simulink model "SignalRouting_Demo"  (R2017b)
settings: Solver=VariableStepAuto  StartTime=0.0  StopTime=10.0  RelTol=1e-3
settings Model: Creator=javed  LastModifiedBy=javed

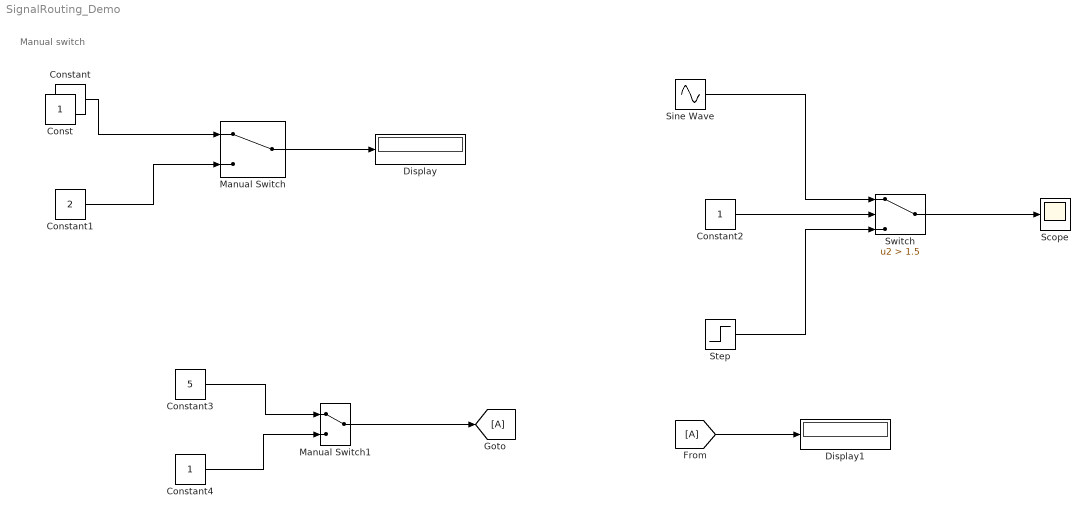
== system SignalRouting_Demo ==
  note: Manual switch
  Constant : Constant  Value=5
  Constant1 : Constant  Value=2
  Constant2 : Constant
  Constant3 : Constant  Value=5
  Constant4 : Constant
  Display : Display
  Display1 : Display
  Manual Switch : ManualSwitch
  Manual Switch1 : ManualSwitch
  Scope : Scope
  Sine Wave : Sin  SampleTime=0
  Step : Step  After=2  SampleTime=0
  Switch : Switch  Criteria=u2 > Threshold  Threshold=1.5
  Const : Constant  IOType=siggen
  wires:
  Manual Switch/1 -> Display/1
  Constant/1 -> Manual Switch/1
  Constant1/1 -> Manual Switch/2
  Constant2/1 -> Switch/2
  Sine Wave/1 -> Switch/1
  Switch/1 -> Scope/1
  Step/1 -> Switch/3
  [A] -> Display1/1
  Manual Switch1/1 -> [A]
  Constant4/1 -> Manual Switch1/2
  Constant3/1 -> Manual Switch1/1
